simulink model "Params_Estimate"  (R2026a)
settings: Solver=ode4  StopTime=60  FixedStep=0.001
values from neighbouring files (symbols this model uses):
  B = 0.001    [create_simu.m]    (also in fix_plot_2.m = 0.19279; motor_grey_ode.m = [1/L_m; 0]; motor_grey_ode_v2.m = [1/L_m; 0]; plot_report_2.m = 0.19279)
  eta = 0.83607    [PID.m]    (also in create_simu.m = 0.85; export_rod.m; fix_plot_2.m; loop_shaping.m)
  J = 0.72762    [PID.m]    (also in create_simu.m = 0.2546; export_rod.m; fix_plot_2.m; loop_shaping.m)
  K_e = 0.04165    [PID.m]    (also in create_simu.m = 0.0321; export_rod.m; fix_plot_2.m; loop_shaping.m)
  K_t = 0.04065    [PID.m]    (also in create_simu.m = 0.0382; export_rod.m; fix_plot_2.m; loop_shaping.m)
  L_m = 0.00144802    [PID.m]    (also in create_simu.m = 0.00147261; export_rod.m; fix_plot_2.m = 0.001448; greybox_sysid.m = 0.00147)
  N_total = 70    [PID.m]    (also in create_simu.m; export_rod.m; fix_plot_2.m; loop_shaping.m)
  R_m = 1.45336    [PID.m]    (also in create_simu.m = 1.53982909; export_rod.m; fix_plot_2.m = 1.4534; greybox_sysid.m = 1.45)
settings Model: Creator=thadzy  LastModifiedBy=thadzy

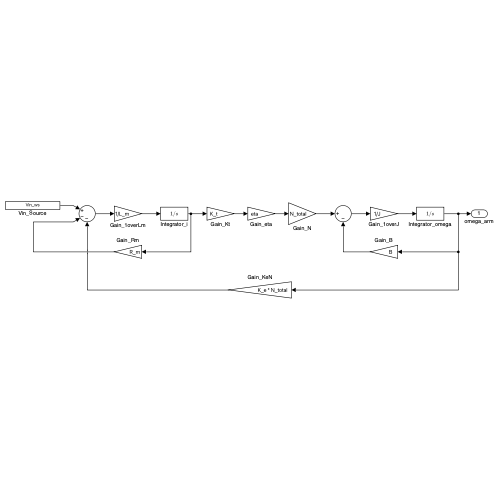
[thumbnail: Simulink's stored preview of the top-level diagram]
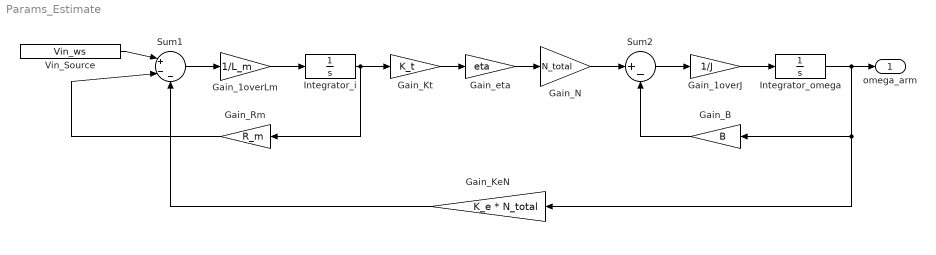
== system Params_Estimate ==
  Gain_1overJ : Gain  Gain=1/J
  Gain_1overLm : Gain  Gain=1/L_m
  Gain_B : Gain  Gain=B
  Gain_KeN : Gain  Gain=K_e * N_total
  Gain_Kt : Gain  Gain=K_t
  Gain_N : Gain  Gain=N_total
  Gain_Rm : Gain  Gain=R_m
  Gain_eta : Gain  Gain=eta
  Integrator_i : Integrator
  Integrator_omega : Integrator
  Sum1 : Sum  Inputs=|+--
  Sum2 : Sum  Inputs=|+-
  Vin_Source : FromWorkspace  VariableName=Vin_ws  SampleTime=0.001
  omega_arm : Outport
  wires:
  Vin_Source/1 -> Sum1/1
  Sum1/1 -> Gain_1overLm/1
  Gain_1overLm/1 -> Integrator_i/1
  Integrator_i/1 -> Gain_Kt/1, Gain_Rm/1
  Gain_Kt/1 -> Gain_eta/1
  Gain_eta/1 -> Gain_N/1
  Gain_N/1 -> Sum2/1
  Gain_Rm/1 -> Sum1/2
  Sum2/1 -> Gain_1overJ/1
  Gain_1overJ/1 -> Integrator_omega/1
  Integrator_omega/1 -> Gain_B/1, Gain_KeN/1, omega_arm/1
  Gain_B/1 -> Sum2/2
  Gain_KeN/1 -> Sum1/3
